simulink model "ros_interface"  (R2019a)
settings: Solver=FixedStepAuto  StartTime=0.0  StopTime=5  FixedStep=0.01  RelTol=1e-3
values from neighbouring files (symbols this model uses):
  Ts = 0.01    [ball_control.m]
undefined symbols (not defined in the file or in its folder): Position
libraries: robotlib x5
settings Model: Creator=nicola  LastModifiedBy=nicola

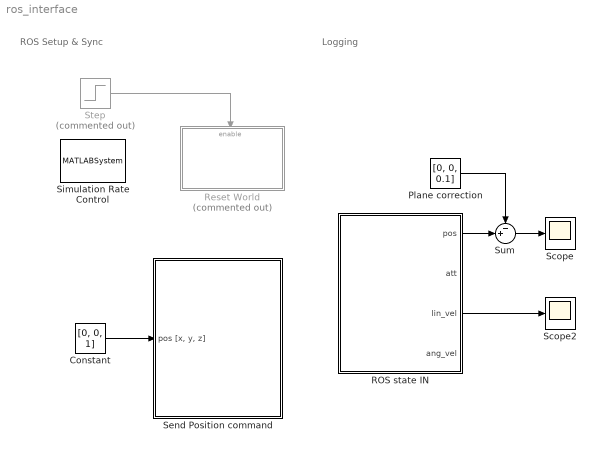
== system ros_interface ==
  note: ROS Setup & Sync
  note: Logging
  Constant : Constant  Value=[0, 0, 1]
  Plane correction : Constant  Value=[0, 0, 0.1]
  ROS state IN : Subsystem
  Reset World : Subsystem  Commented=on
  Scope : Scope
  Scope2 : Scope
  Send Position command : Subsystem
  Simulation Rate Control : MATLABSystem  System=ExampleHelperSimulationRateControl  SampleTime=Ts*2
      mask Type: ExampleHelperSimulationRateControl
      mask Display: disp('Rate Control');
  Step : Step  Commented=on  Time=1 * Ts  Before=1  After=0
  Sum : Sum  Inputs=-+|
  wires:
  Step/1 -> Reset World/Enable
  Constant/1 -> Send Position command/1("pos [x, y, z]")
  ROS state IN/1(pos) -> Sum/2
  ROS state IN/3(lin_vel) -> Scope2/1
  Sum/1 -> Scope/1
  Plane correction/1 -> Sum/1

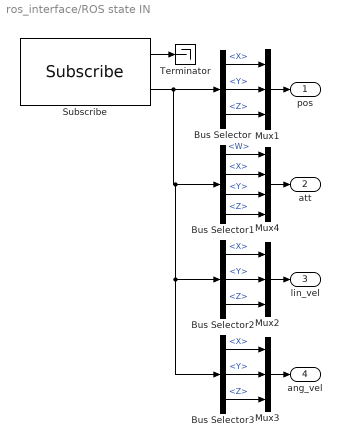
== system ros_interface/ROS state IN ==
  Bus Selector : BusSelector  OutputSignals=Pose.Pose.Position.X,Pose.Pose.Position.Y,Pose.Pose.Position.Z
  Bus Selector1 : BusSelector  OutputSignals=Pose.Pose.Orientation.W,Pose.Pose.Orientation.X,Pose.Pose.Orientation.Y,Pose.Pose.Orientation.Z
  Bus Selector2 : BusSelector  OutputSignals=Twist.Twist.Linear.X,Twist.Twist.Linear.Y,Twist.Twist.Linear.Z
  Bus Selector3 : BusSelector  OutputSignals=Twist.Twist.Angular.X,Twist.Twist.Angular.Y,Twist.Twist.Angular.Z
  Mux1 : Mux  Inputs=3
  Mux2 : Mux  Inputs=3
  Mux3 : Mux  Inputs=3
  Mux4 : Mux
  Subscribe : robotlib/Subscribe  topicSource=Select from ROS network  topic=/force_control/odometry  messageType=nav_msgs/Odometry  sampleTime=-1  messageQueueLength=1
      settings: SourceProductBaseCode=RO
  Terminator : Terminator
  pos : Outport
  att : Outport  Port=2
  lin_vel : Outport  Port=3
  ang_vel : Outport  Port=4
  wires:
  Bus Selector3/2 -> Mux3/2  "<Y>"
  Bus Selector/2 -> Mux1/2  "<Y>"
  Bus Selector/1 -> Mux1/1  "<X>"
  Bus Selector/3 -> Mux1/3  "<Z>"
  Mux2/1 -> lin_vel/1
  Bus Selector2/1 -> Mux2/1  "<X>"
  Subscribe/1 -> Terminator/1
  Bus Selector1/2 -> Mux4/2  "<X>"
  Bus Selector3/1 -> Mux3/1  "<X>"
  Bus Selector1/4 -> Mux4/4  "<Z>"
  Bus Selector1/3 -> Mux4/3  "<Y>"
  Mux3/1 -> ang_vel/1
  Subscribe/2 -> Bus Selector3/1, Bus Selector2/1, Bus Selector1/1, Bus Selector/1
  Mux1/1 -> pos/1
  Bus Selector1/1 -> Mux4/1  "<W>"
  Bus Selector3/3 -> Mux3/3  "<Z>"
  Bus Selector2/3 -> Mux2/3  "<Z>"
  Mux4/1 -> att/1
  Bus Selector2/2 -> Mux2/2  "<Y>"

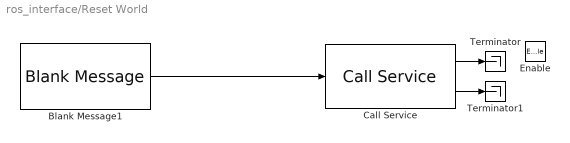
== system ros_interface/Reset World ==
  Enable : EnablePort  StatesWhenEnabling=reset
  Blank Message1 : robotlib/Blank Message  messageClass=Service Request  entityType=std_srvs/Empty  messageType=std_srvs/EmptyRequest  SampleTime=inf
      settings: SourceProductBaseCode=RO
  Call Service : robotlib/Call Service  topicSource=Select from ROS network  service=/gazebo/reset_world  serviceType=std_srvs/Empty  connectionTimeout=5  keepPersistent=off  ShowErrorCodeOutput=on
      settings: SourceProductName=Robotics System Toolbox  SourceProductBaseCode=RO
  Terminator : Terminator
  Terminator1 : Terminator
  wires:
  Call Service/1 -> Terminator/1
  Call Service/2 -> Terminator1/1
  Blank Message1/1 -> Call Service/1

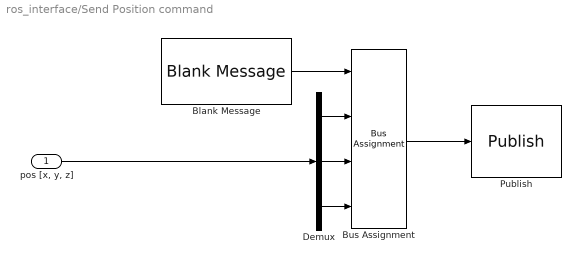
== system ros_interface/Send Position command ==
  "pos [x, y, z]" : Inport
  Blank Message : robotlib/Blank Message  messageClass=Message  entityType=geometry_msgs/Pose  messageType=geometry_msgs/Pose  SampleTime=inf
      settings: SourceProductBaseCode=RO
  Bus Assignment : BusAssignment  AssignedSignals=Position.X,Position.Y,Position.Z
  Demux : Demux  Outputs=3
  Publish : robotlib/Publish  topicSource=Select from ROS network  topic=/force_control/command/position  messageType=geometry_msgs/Pose  messageQueueLength=1
      settings: SourceProductBaseCode=RO
  wires:
  Blank Message/1 -> Bus Assignment/1
  Bus Assignment/1 -> Publish/1
  Demux/1 -> Bus Assignment/2
  Demux/2 -> Bus Assignment/3
  "pos [x, y, z]"/1 -> Demux/1
  Demux/3 -> Bus Assignment/4
